simulink model "StabilityControlSystemRestructured"  (R2023a)
settings: Solver=VariableStepAuto  StartTime=0.0  StopTime=10.0  RelTol=1e-3
libraries: simulink x2, slpidlib x1
settings Model: Creator=edill  LastModifiedBy=harshs
settings RTWCC: GPUComputeCapability=5.0
settings ConfigComp: CovBoundaryAbsTol=1.0e-5

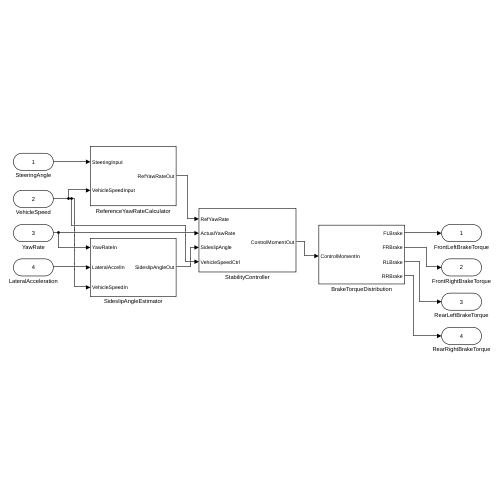
[thumbnail: Simulink's stored preview of the top-level diagram]
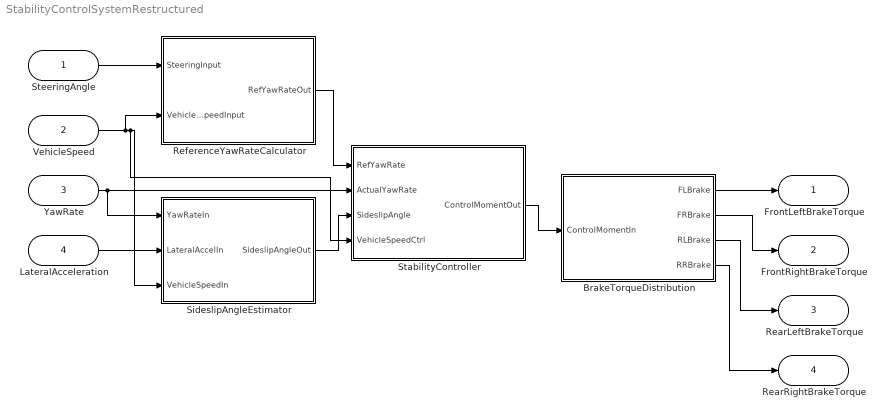
== system StabilityControlSystemRestructured ==
  SteeringAngle : Inport
  VehicleSpeed : Inport  Port=2
  YawRate : Inport  Port=3
  LateralAcceleration : Inport  Port=4
  BrakeTorqueDistribution : Subsystem
  ReferenceYawRateCalculator : Subsystem
  SideslipAngleEstimator : Subsystem
  StabilityController : Subsystem
  FrontLeftBrakeTorque : Outport
  FrontRightBrakeTorque : Outport  Port=2
  RearLeftBrakeTorque : Outport  Port=3
  RearRightBrakeTorque : Outport  Port=4
  wires:
  SideslipAngleEstimator/1(SideslipAngleOut) -> StabilityController/3(SideslipAngle)
  SteeringAngle/1 -> ReferenceYawRateCalculator/1(SteeringInput)
  VehicleSpeed/1 -> SideslipAngleEstimator/3(VehicleSpeedIn), StabilityController/4(VehicleSpeedCtrl), ReferenceYawRateCalculator/2(VehicleSpeedInput)
  BrakeTorqueDistribution/1(FLBrake) -> FrontLeftBrakeTorque/1
  YawRate/1 -> StabilityController/2(ActualYawRate), SideslipAngleEstimator/1(YawRateIn)
  LateralAcceleration/1 -> SideslipAngleEstimator/2(LateralAccelIn)
  ReferenceYawRateCalculator/1(RefYawRateOut) -> StabilityController/1(RefYawRate)
  StabilityController/1(ControlMomentOut) -> BrakeTorqueDistribution/1(ControlMomentIn)
  BrakeTorqueDistribution/2(FRBrake) -> FrontRightBrakeTorque/1
  BrakeTorqueDistribution/3(RLBrake) -> RearLeftBrakeTorque/1
  BrakeTorqueDistribution/4(RRBrake) -> RearRightBrakeTorque/1

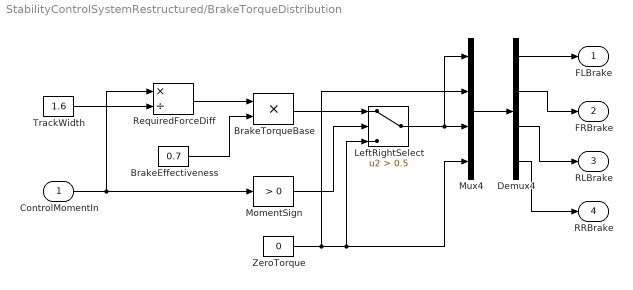
== system StabilityControlSystemRestructured/BrakeTorqueDistribution ==
  ControlMomentIn : Inport
  BrakeEffectiveness : Constant  Value=0.7
  BrakeTorqueBase : Product
  Demux4 : Demux
  LeftRightSelect : Switch  Criteria=u2 > Threshold  Threshold=0.5  SaturateOnIntegerOverflow=off  InputSameDT=off
  MomentSign : simulink/Logic and Bit Operations/Compare To Zero  relop=>  OutDataTypeStr=boolean
  Mux4 : Mux
  RequiredForceDiff : Product  Inputs=*/
  TrackWidth : Constant  Value=1.6
  ZeroTorque : Constant  Value=0
  FLBrake : Outport
  FRBrake : Outport  Port=2
  RLBrake : Outport  Port=3
  RRBrake : Outport  Port=4
  wires:
  Demux4/3 -> RLBrake/1
  TrackWidth/1 -> RequiredForceDiff/2
  ControlMomentIn/1 -> MomentSign/1, RequiredForceDiff/1
  RequiredForceDiff/1 -> BrakeTorqueBase/1
  BrakeEffectiveness/1 -> BrakeTorqueBase/2
  LeftRightSelect/1 -> Mux4/1, Mux4/3
  MomentSign/1 -> LeftRightSelect/2
  BrakeTorqueBase/1 -> LeftRightSelect/1
  ZeroTorque/1 -> Mux4/4, LeftRightSelect/3, Mux4/2
  Mux4/1 -> Demux4/1
  Demux4/1 -> FLBrake/1
  Demux4/2 -> FRBrake/1
  Demux4/4 -> RRBrake/1

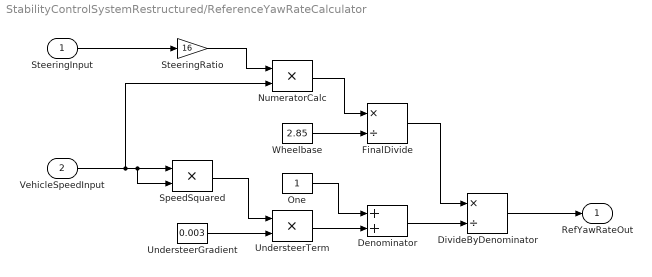
== system StabilityControlSystemRestructured/ReferenceYawRateCalculator ==
  SteeringInput : Inport
  VehicleSpeedInput : Inport  Port=2
  Denominator : Sum
  DivideByDenominator : Product  Inputs=*/
  FinalDivide : Product  Inputs=*/
  NumeratorCalc : Product
  One : Constant
  SpeedSquared : Product
  SteeringRatio : Gain  Gain=16
  UndersteerGradient : Constant  Value=0.003
  UndersteerTerm : Product
  Wheelbase : Constant  Value=2.85
  RefYawRateOut : Outport
  wires:
  VehicleSpeedInput/1 -> SpeedSquared/2, SpeedSquared/1, NumeratorCalc/2
  SteeringInput/1 -> SteeringRatio/1
  SteeringRatio/1 -> NumeratorCalc/1
  One/1 -> Denominator/1
  SpeedSquared/1 -> UndersteerTerm/1
  NumeratorCalc/1 -> FinalDivide/1
  UndersteerGradient/1 -> UndersteerTerm/2
  Wheelbase/1 -> FinalDivide/2
  UndersteerTerm/1 -> Denominator/2
  FinalDivide/1 -> DivideByDenominator/1
  Denominator/1 -> DivideByDenominator/2
  DivideByDenominator/1 -> RefYawRateOut/1

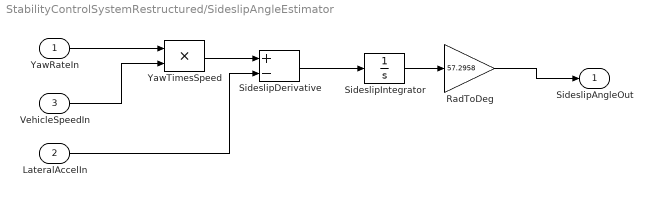
== system StabilityControlSystemRestructured/SideslipAngleEstimator ==
  YawRateIn : Inport
  LateralAccelIn : Inport  Port=2
  VehicleSpeedIn : Inport  Port=3
  RadToDeg : Gain  Gain=57.2958
  SideslipDerivative : Sum  Inputs=+-
  SideslipIntegrator : Integrator
  YawTimesSpeed : Product
  SideslipAngleOut : Outport
  wires:
  YawTimesSpeed/1 -> SideslipDerivative/1
  SideslipDerivative/1 -> SideslipIntegrator/1
  SideslipIntegrator/1 -> RadToDeg/1
  LateralAccelIn/1 -> SideslipDerivative/2
  YawRateIn/1 -> YawTimesSpeed/1
  RadToDeg/1 -> SideslipAngleOut/1
  VehicleSpeedIn/1 -> YawTimesSpeed/2

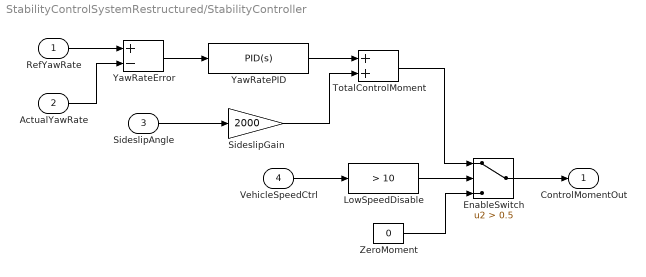
== system StabilityControlSystemRestructured/StabilityController ==
  RefYawRate : Inport
  ActualYawRate : Inport  Port=2
  SideslipAngle : Inport  Port=3
  VehicleSpeedCtrl : Inport  Port=4
  EnableSwitch : Switch  Criteria=u2 > Threshold  Threshold=0.5  SaturateOnIntegerOverflow=off  InputSameDT=off
  LowSpeedDisable : simulink/Logic and Bit Operations/Compare To Constant  relop=>  const=10  OutDataTypeStr=boolean
  SideslipGain : Gain  Gain=2000
  TotalControlMoment : Sum
  YawRateError : Sum  Inputs=+-
  YawRatePID : slpidlib/PID Controller  Controller=PID  Form=Parallel  TimeDomain=Continuous-time  UseExternalTs=off  SampleTime=-1  IntegratorMethod=Forward Euler  FilterMethod=Forward Euler  ControllerParametersSource=internal  P=5000  I=1000  UseKiTs=off  D=100  N=100  UseFilter=on  TunerSelectOption=Transfer Function Based (PID Tuner App)  InitialConditionSource=internal  InitialConditionForIntegrator=0  InitialConditionForFilter=0  DifferentiatorICPrevScaledInput=0  ExternalReset=none  TrackingMode=off  Kt=1  LimitOutput=off  SatLimitsSource=internal  UpperSaturationLimit=inf  LowerSaturationLimit=-inf  LinearizeAsGain=on  AntiWindupMode=none  Kb=1  LimitIntegrator=off  UpperIntegratorSaturationLimit=inf  LowerIntegratorSaturationLimit=-inf  POutMin=[]  POutMax=[]  IOutMin=[]  IOutMax=[]  DOutMin=[]  DOutMax=[]  NOutMin=[]  NOutMax=[]  SumOutMin=[]  SumOutMax=[]  SaturationOutMin=[]  SaturationOutMax=[]  PParamMin=[]  PParamMax=[]  IParamMin=[]  IParamMax=[]  DParamMin=[]  DParamMax=[]  NParamMin=[]  NParamMax=[]  KbParamMin=[]  KbParamMax=[]  KtParamMin=[]  KtParamMax=[]  KbOutMin=[]  KbOutMax=[]  KtOutMin=[]  KtOutMax=[]  IntegratorOutMin=[]  IntegratorOutMax=[]  FilterOutMin=[]  FilterOutMax=[]  SumI1OutMin=[]  SumI1OutMax=[]  SumI2OutMin=[]  SumI2OutMax=[]  SumI3OutMin=[]  SumI3OutMax=[]  SumI4OutMin=[]  SumI4OutMax=[]  SumDOutMin=[]  SumDOutMax=[]  DifferentiatorOutMin=[]  DifferentiatorOutMax=[]  FilterDiffOutCoefMin=[]  FilterDiffOutCoefMax=[]  ReciprocalOutMin=[]  ReciprocalOutMax=[]  SumDenOutMin=[]  SumDenOutMax=[]  SumNumOutMin=[]  SumNumOutMax=[]  DivideOutMin=[]  DivideOutMax=[]  UdiffTsProdOutMin=[]  UdiffTsProdOutMax=[]  NTsProdOutMin=[]  NTsProdOutMax=[]  UintegralTsProdOutMin=[]  UintegralTsProdOutMax=[]  UngainTsProdOutMin=[]  UngainTsProdOutMax=[]  ClampingZeroOutDataTypeStr=Inherit: Inherit via back propagation  ClampingZeroOutMin=[]  ClampingZeroOutMax=[]  FilterDenConstantOutDataTypeStr=Inherit: Inherit via back propagation  FilterDenConstantOutMin=[]  FilterDenConstantOutMax=[]  PCopyOutDataTypeStr=Inherit: Inherit via back propagation  PCopyOutMin=[]  PCopyOutMax=[]  NCopyOutDataTypeStr=Inherit: Inherit via back propagation  NCopyOutMin=[]  NCopyOutMax=[]  IntegratorContinuousStateAttributes=''  IntegratorStateMustResolveToSignalObject=off  IntegratorRTWStateStorageClass=Auto  FilterContinuousStateAttributes=''  FilterStateMustResolveToSignalObject=off  FilterRTWStateStorageClass=Auto  ParallelPVariant=InternalParameters  IdealPVariant=Disabled  IVariant=InternalParameters  DVariant=InternalParameters  IntegratorVariant=Continuous  SatVariant=Disabled  AWVariant=Passthrough  PCopyVariant=Disabled  TRVariant=Disabled  FdbkBlocksVariant=Forward  IdealPFdbkVariant=Disabled  SatFdbkVariant=Disabled  DerivativeFilterVariant=ContFilter  NVariant=InternalParameters  NCopyVariant=Disabled  FilterICVariant=InternalICsFilter  IntegratorICVariant=InternalICs  ExternalResetVariant=Disabled  TRSumVariant=Passthrough  SumFdbkVariant=Disabled  SumVariant=Sum_PID  TsampFilterVariant=InternalTs  TsampNgainVariant=Passthrough  TsampIntegralVariant=Disabled_SignalSpec  ExternalSaturationOutDataTypeStr=Inherit: Same as second input
  ZeroMoment : Constant  Value=0
  ControlMomentOut : Outport
  wires:
  RefYawRate/1 -> YawRateError/1
  VehicleSpeedCtrl/1 -> LowSpeedDisable/1
  YawRatePID/1 -> TotalControlMoment/1
  YawRateError/1 -> YawRatePID/1
  ActualYawRate/1 -> YawRateError/2
  SideslipAngle/1 -> SideslipGain/1
  SideslipGain/1 -> TotalControlMoment/2
  TotalControlMoment/1 -> EnableSwitch/1
  LowSpeedDisable/1 -> EnableSwitch/2
  ZeroMoment/1 -> EnableSwitch/3
  EnableSwitch/1 -> ControlMomentOut/1
